simulink model "filter_low_high"  (R2021a)
settings: Solver=FixedStepAuto  StartTime=0.0  StopTime=50  FixedStep=0.01  RelTol=1e-3
settings Model: Creator=admin  LastModifiedBy=admin

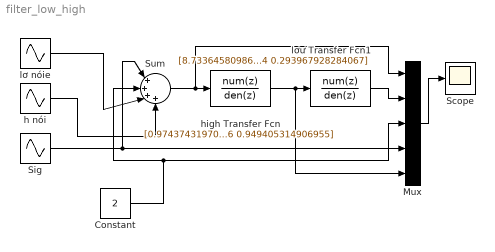
== system filter_low_high ==
  Constant : Constant  Value=2
  Mux : Mux  Inputs=5
  Scope : Scope
  Sig : Sin  Frequency=2*pi*1.5  SampleTime=0.01
  Sum : Sum  Inputs=|++++
  h nói : Sin  Amplitude=4  Frequency=2*pi*50  SampleTime=0.01
  high Transfer Fcn : DiscreteTransferFcn  Numerator=[0.974374319708270 -3.897497278833082 5.846245918249623 -3.897497278833082 0.974374319708270]  Denominator=[1 -3.948081940141342 5.845589318686745 -3.846912541597286 0.949405314906955]
  lơ nóie : Sin  Amplitude=2  Frequency=2*pi*0.05  SampleTime=0.01
  lơư Transfer Fcn1 : DiscreteTransferFcn  Numerator="[8.73364580986315e-06\t5.24018748591789e-05\t0.000131004687147947\t0.000174672916197263\t0.000131004687147947 5.24018748591789e-05\t8.73364580986315e-06]"  Denominator=[1 -4.783119805467426 9.634103030016156 -10.445088376732409 6.422227494861858 -2.121531317630414 0.293967928284067]
  wires:
  high Transfer Fcn/1 -> Mux/5, lơư Transfer Fcn1/1
  Mux/1 -> Scope/1
  lơư Transfer Fcn1/1 -> Mux/2
  Constant/1 -> Sum/2, Mux/3
  Sum/1 -> Mux/1, high Transfer Fcn/1
  Sig/1 -> Mux/4, Sum/1
  lơ nóie/1 -> Sum/3
  h nói/1 -> Sum/4
